simulink model "analog_differentiator"  (R2020b)
settings: Solver=ode1be  StartTime=0.0  StopTime=10  RelTol=1e-3  AbsTol=1e-3
libraries: analogCompBlocks x3, fl_lib x1, ee_lib x1, nesl_utility x1
settings Model: DataDictionary=analogComputerData.sldd  EnableAccessToBaseWorkspace=off  OrderedModelArguments=off  Creator=roadrunner  LastModifiedBy=roadrunner
settings SolverCC: AutoScaleAbsTol=off
settings DebuggingCC: SymbolicDimsDataTypeCodeGenerationDiagnostic=none
settings SFSimCC: CustomCodeUndefinedFunction=UseInterfaceOnly
settings SimscapeCC: SimscapeLogType=all  SimscapeLogSimulationStatistics=on  SimscapeLogDataHistory=10000

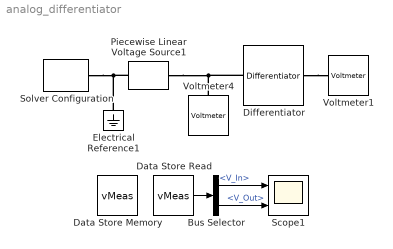
== system analog_differentiator ==
  Bus Selector : BusSelector  OutputSignals=V_In,V_Out
  Data Store Memory : DataStoreMemory  Priority=5  DataStoreName=vMeas  ReadBeforeWriteMsg=warning  WriteAfterWriteMsg=warning  WriteAfterReadMsg=warning  ShowAdditionalParam=off  OutDataTypeStr=Bus: bus_differentiator_measurements
  Data Store Read : DataStoreRead  Priority=6  DataStoreName=vMeas
  Differentiator : analogCompBlocks/Differentiator  capacitance=0.1  tau=1
  Electrical Reference1 : fl_lib/Electrical/Electrical Elements/Electrical Reference
  Piecewise Linear Voltage Source1 : ee_lib/Additional Components/SPICE Sources/Piecewise Linear Voltage Source  TIMElist=[2 5 8] s  VOLTlist=[0 3 0] V  INTERP=1  EXTRAP=2
      settings: AttributesFormatString=Voltage In  SourceProductBaseCode=PS  InternalSimscapePortConfiguration="{\"Bottom\":[],\"Left\":[{\"id\":\"p\",\"label\":\"+\",\"type\":\"foundation.electrical.electrical\"}],\"Right\":[{\"id\":\"n\",\"label\":\"-\",\"type\":\"foundation.electrical.electrical\"}],\"Top\":[]}"
  Scope1 : Scope  NumInputPorts=2
  Solver Configuration : nesl_utility/Solver Configuration  PhysicalDomain=network_engine_domain  SubClassName=solver  LeftPortType=input  RightPortType=generic  Tones=[]  Harmonics=[]  SimulateNoise=off  Profile=off  UseLocalSampling=off  EnableSwitchedLinearOptims=on  FrequencyDomain=off  UseCCode=off  RelTol=0.001  AbsTol=1e-06  MinStep=1e-09  ToWorkspace=off  RevertToSquareIcSolve=off  NumHomotopyIterations=100  PhasorMode=off  PhasorModeNumHarmonics=1  DoDC=off  ResidualTolerance=1e-09  UseLocalSolver=on  LocalSolverChoice=NE_BACKWARD_EULER_ADVANCER  LocalSolverSampleTime=0.01  DoFixedCost=on  MaxNonlinIter=3  MaxModeIter=2  ComputeImpulses=off  ImpulseIterations=2  LinearAlgebra=auto  EquationFormulation=NE_TIME_EF  DelaysMemoryBudget=1024  AutomaticFiltering=on  FilteringTimeConstant=0.001  PartitionStorageMethod=AS_NEEDED  PartitionMemoryBudget=1024  PartitionMethod=ROBUST
      settings: SourceProductName=Utilities
  Voltmeter1 : analogCompBlocks/Voltmeter  Priority=4  DSNAME='vMeas'  DSELEMENT='V_Out'
      settings: AttributesFormatString=Voltage Sensor
  Voltmeter4 : analogCompBlocks/Voltmeter  Priority=2  DSNAME='vMeas'  DSELEMENT='V_In'
      settings: AttributesFormatString=Voltage Sensor
  wires:
  Data Store Read/1 -> Bus Selector/1
  Bus Selector/1 -> Scope1/1  "<V_In>"
  Bus Selector/2 -> Scope1/2  "<V_Out>"
  connections:
  Electrical Reference1/LConn1 -- Piecewise Linear Voltage Source1/RConn1 -- Solver Configuration/RConn1
  Piecewise Linear Voltage Source1/LConn1 -- Differentiator/LConn1 -- Voltmeter4/LConn1
  Differentiator/RConn1 -- Voltmeter1/LConn1
